simulink model "prob7_model"  (R2020a)
settings: Solver=VariableStepAuto  StartTime=0.0  StopTime=10.0  RelTol=1e-3
settings Model: Creator=sonal  LastModifiedBy=sonal
settings DataIOCC: SaveOutput=off  SaveTime=off

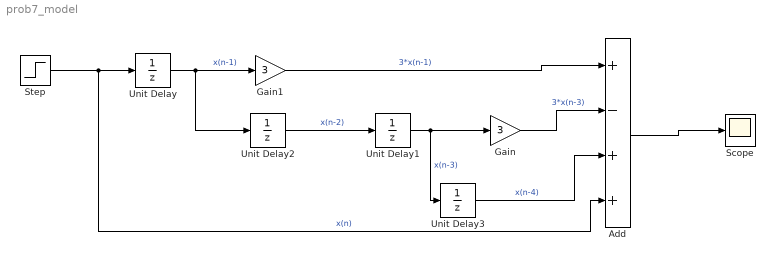
== system prob7_model ==
  Add : Sum  Inputs=+-++
  Gain : Gain  Gain=3
  Gain1 : Gain  Gain=3
  Scope : Scope
  Step : Step  SampleTime=0
  Unit Delay{,1..3} (4 alike) : UnitDelay  SampleTime=-1  HasFrameUpgradeWarning=on
  wires:
  Unit Delay3/1 -> Add/3  "x(n-4)"
  Gain/1 -> Add/2  "3*x(n-3)"
  Unit Delay/1 -> Gain1/1, Unit Delay2/1  "x(n-1)"
  Add/1 -> Scope/1
  Unit Delay1/1 -> Gain/1, Unit Delay3/1  "x(n-3)"
  Step/1 -> Unit Delay/1, Add/4  "x(n)"
  Unit Delay2/1 -> Unit Delay1/1  "x(n-2)"
  Gain1/1 -> Add/1  "3*x(n-1)"
